simulink model "tdm_pcm"  (R2018a)
settings: Solver=VariableStepAuto  StartTime=0.0  StopTime=10.0  RelTol=1e-3
libraries: commutil2 x2, dspquant2 x2, simulink_extras x1, dspsigops x1, dsparch4 x1
settings Model: Creator=hp  LastModifiedBy=hp

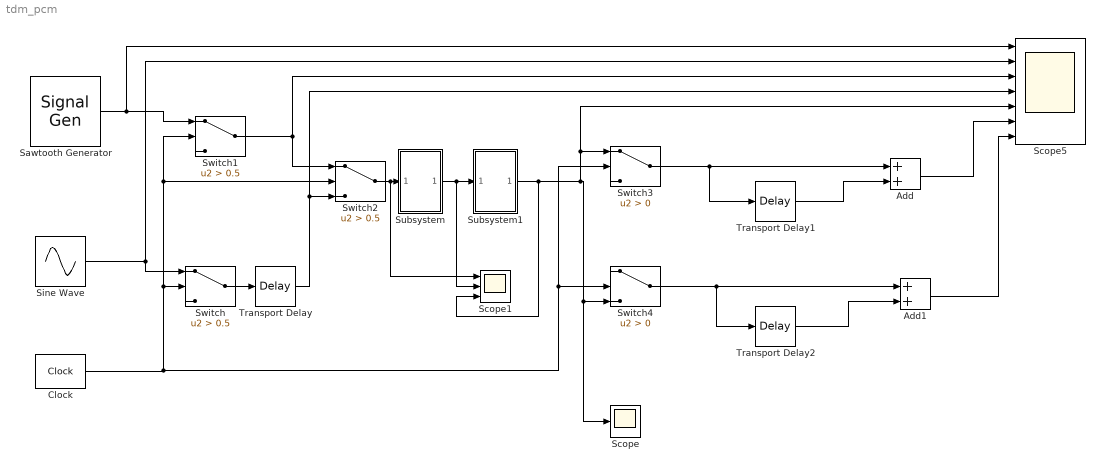
== system tdm_pcm ==
  Add : Sum
  Add1 : Sum
  Clock : simulink_extras/Flip Flops/Clock  period=2
  Sawtooth Generator : SignalGenerator  WaveForm=sawtooth  Amplitude=4  Frequency=4
  Scope : Scope
  Scope1 : Scope  NumInputPorts=3
  Scope5 : Scope  NumInputPorts=7
  Sine Wave : Sin  Amplitude=2  Frequency=2*pi*1  SampleTime=0.01
  Subsystem : Subsystem
  Subsystem1 : Subsystem
  Switch : Switch  Criteria=u2 > Threshold  Threshold=0.5
  Switch1 : Switch  Criteria=u2 > Threshold  Threshold=0.5
  Switch2 : Switch  Criteria=u2 > Threshold  Threshold=0.5
  Switch3 : Switch  Criteria=u2 > Threshold
  Switch4 : Switch  Criteria=u2 > Threshold
  Transport Delay : TransportDelay
  Transport Delay1 : TransportDelay
  Transport Delay2 : TransportDelay
  wires:
  Switch3/1 -> Transport Delay1/1, Add/1
  Add1/1 -> Scope5/7
  Switch/1 -> Transport Delay/1
  Switch1/1 -> Scope5/3, Switch2/1
  Transport Delay1/1 -> Add/2
  Sawtooth Generator/1 -> Scope5/1, Switch1/1
  Transport Delay2/1 -> Add1/2
  Switch4/1 -> Transport Delay2/1, Add1/1
  Sine Wave/1 -> Switch/1, Scope5/2
  Clock/1 -> Switch4/2, Switch3/2, Switch1/2, Switch2/2, Switch/2
  Add/1 -> Scope5/6
  Transport Delay/1 -> Scope5/4, Switch2/3
  Switch2/1 -> Scope1/1, Subsystem/1(In1)
  Subsystem1/1(Out1) -> Scope1/3, Scope/1, Switch4/3, Scope5/5, Switch3/1
  Subsystem/1(Out1) -> Scope1/2, Subsystem1/1(In1)

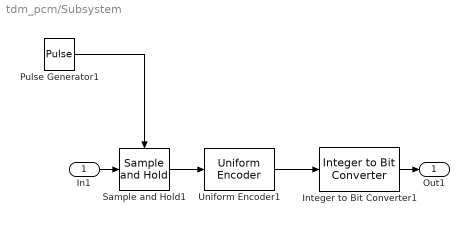
== system tdm_pcm/Subsystem ==
  In1 : Inport
  Integer to Bit Converter1 : commutil2/Integer to Bit Converter  nbits=3  signedInputValues=Unsigned  bitOrder=MSB first  outDtype=Inherit via internal rule
  Pulse Generator1 : DiscretePulseGenerator  PulseType=Time based  Period=1/30  PulseWidth=50
  Sample and Hold1 : dspsigops/Sample and Hold  trig=Rising edge  initCond=0  latchinput=off
  Uniform Encoder1 : dspquant2/Uniform Encoder  peak=5  bits=3  otype=Unsigned integer
      settings: SourceProductName=DSP System Toolbox
  Out1 : Outport
  wires:
  Pulse Generator1/1 -> Sample and Hold1/Trigger
  In1/1 -> Sample and Hold1/1
  Uniform Encoder1/1 -> Integer to Bit Converter1/1
  Sample and Hold1/1 -> Uniform Encoder1/1
  Integer to Bit Converter1/1 -> Out1/1

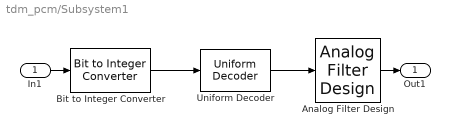
== system tdm_pcm/Subsystem1 ==
  In1 : Inport
  Analog Filter Design : dsparch4/Analog Filter Design  method=Butterworth  filttype=Lowpass  N=2  Wlo=2*pi*1  Whi=80  Rp=2  Rs=40
  Bit to Integer Converter : commutil2/Bit to Integer Converter  nbits=3  bitOrder=MSB first  signedOutputValues=Unsigned  outDtype=Inherit via internal rule  outDtypeSigned=Inherit via internal rule
  Uniform Decoder : dspquant2/Uniform Decoder  peak=5  bits=3  overflowMode=Saturate  otype=Double
      settings: SourceProductName=DSP System Toolbox  SourceProductBaseCode=DS
  Out1 : Outport
  wires:
  Uniform Decoder/1 -> Analog Filter Design/1
  Bit to Integer Converter/1 -> Uniform Decoder/1
  Analog Filter Design/1 -> Out1/1
  In1/1 -> Bit to Integer Converter/1
